simulink subsystem "Visualization"  (R2020a)
settings: Solver=VariableStepAuto  StartTime=0.0  StopTime=10.0  RelTol=1e-3
settings Model: Creator=frede  LastModifiedBy=zinoex

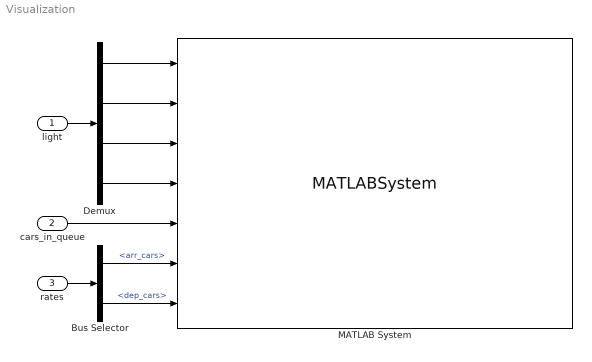
== system Visualization ==
  light : Inport
  cars_in_queue : Inport  Port=2
  rates : Inport  Port=3
  Bus Selector : BusSelector  OutputSignals=arr_cars,dep_cars
  Demux : Demux
  MATLAB System : MATLABSystem  System=IntersectionPlotter
      mask Type: IntersectionPlotter
      mask Display:
      | disp('IntersectionPlotter');
      | port_label('input',1,'Green');
      | port_label('input',2,'Red');
      | port_label('input',3,'Yellow');
      | port_label('input',4,'Amber');
      | port_label('input',5,'QueueSizes');
      | port_label('input',6,'ArrRates');
      | port_label('input',7,'DepRates');
  wires:
  cars_in_queue/1 -> MATLAB System/5
  Bus Selector/1 -> MATLAB System/6  "<arr_cars>"
  Bus Selector/2 -> MATLAB System/7  "<dep_cars>"
  rates/1 -> Bus Selector/1
  light/1 -> Demux/1
  Demux/1 -> MATLAB System/1
  Demux/2 -> MATLAB System/2
  Demux/3 -> MATLAB System/3
  Demux/4 -> MATLAB System/4
